simulink model "proba_sil"  (Simulink 7.7)
settings: Solver=ode45  StartTime=0.0  StopTime=100  RelTol=1e-3
settings Model: Creator=Maciek  LastModifiedBy=Maciek

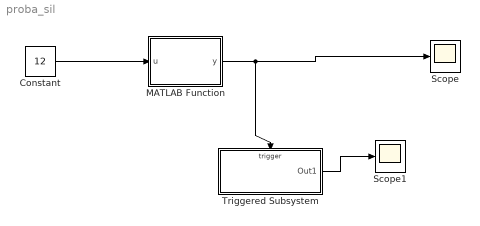
== system proba_sil ==
  Constant : Constant  Value=12
  MATLAB Function : Stateflow chart  TreatAsAtomicUnit=on
  Scope : Scope
      settings: YMin=1200  YMax=1200
  Scope1 : Scope
  Triggered Subsystem : Subsystem  TreatAsAtomicUnit=on
  wires:
  Constant/1 -> MATLAB Function/1(u)
  MATLAB Function/1(y) -> Scope/1, Triggered Subsystem/Trigger
  Triggered Subsystem/1(Out1) -> Scope1/1

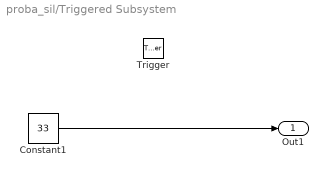
== system proba_sil/Triggered Subsystem ==
  Trigger : TriggerPort
  Constant1 : Constant  Value=33
  Out1 : Outport
  wires:
  Constant1/1 -> Out1/1

== matlab function MATLAB Function ==
  data: u input double; y output double
function y = fcn(u)
%#codegen
coder.extrinsic('pause');
pause(3);
u = u *100;
y = u;
